simulink model "sim_explicit_IC_nonlinear"  (R2020b)
settings: Solver=VariableStepAuto  StartTime=0.0  StopTime=tsim  RelTol=1e-3
values from neighbouring files (symbols this model uses):
  g = 9.81    [init_sim.m]
  m = 0.03    [init_sim.m]
  Ts = 1e-2    (= 0.01)    [init_sim.m]
  u_max = [f_max; tau_max]    [init_sim.m]
  u_min = [f_min; tau_min]    [init_sim.m]
  x0 = zeros(6,1)    [get_sim_data.m]    (also in get_sim_data_mpc_phi.m; get_sim_data_mpc_y.m; get_sim_data_mpc_z.m; init_sim.m = 0.9*[InvSet_y.V(i,1)'; InvSet_z.V(j,1)'; InvSet_phi.V(k,1)';)
  x_max = [y_max;z_max;angle_max;vy_max;vz_max;arate_max]    [init_sim.m]
  x_min = [y_min;z_min;angle_min;vy_min;vz_min;arate_min]    [init_sim.m]
undefined symbols (not defined in the file or in its folder): pid_att, quad_ic_y, quad_ic_z, uavPlanarNonlin
libraries: pid_lib x1
settings Model: SimulationMode=accelerator  Creator=zboucek  LastModifiedBy=zboucek
settings DataIOCC: ReturnWorkspaceOutputs=off
settings DebuggingCC: ArithmeticOperatorsInVariantConditions=warning
settings SFSimCC: SimUseLocalCustomCode=off  CustomCodeUndefinedFunction=UseInterfaceOnly
settings RTWCC: RTWUseLocalCustomCode=off

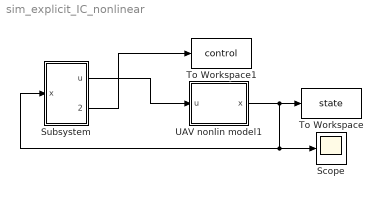
== system sim_explicit_IC_nonlinear ==
  Scope : Scope
  Subsystem : Subsystem
  To Workspace : ToWorkspace  VariableName=state  SaveFormat=Structure With Time  SampleTime=Ts
  To Workspace1 : ToWorkspace  VariableName=control  SaveFormat=Structure With Time  SampleTime=Ts
  UAV nonlin model1 : Subsystem
  wires:
  UAV nonlin model1/1(x) -> Scope/1, Subsystem/1(x), To Workspace/1
  Subsystem/1(u) -> UAV nonlin model1/1(u)
  Subsystem/2(u_ctrl) -> To Workspace1/1

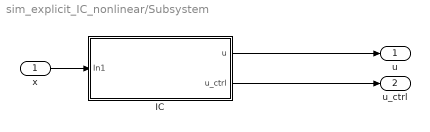
== system sim_explicit_IC_nonlinear/Subsystem ==
  x : Inport
  IC : Subsystem
  u : Outport  VectorParamsAs1DForOutWhenUnconnected=off
  u_ctrl : Outport  Port=2  VectorParamsAs1DForOutWhenUnconnected=off
  wires:
  x/1 -> IC/1(In1)
  IC/1(u) -> u/1
  IC/2(u_ctrl) -> u_ctrl/1

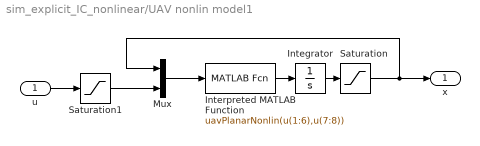
== system sim_explicit_IC_nonlinear/UAV nonlin model1 ==
  u : Inport
  Integrator : Integrator  InitialCondition=x0
  Interpreted MATLAB Function : MATLABFcn  MATLABFcn=uavPlanarNonlin(u(1:6),u(7:8))  OutputDimensions=6
  Mux : Mux  Inputs=2
  Saturation : Saturate  UpperLimit=x_max  LowerLimit=x_min
  Saturation1 : Saturate  UpperLimit=u_max  LowerLimit=u_min
  x : Outport  VectorParamsAs1DForOutWhenUnconnected=off
  wires:
  Mux/1 -> Interpreted MATLAB Function/1
  Interpreted MATLAB Function/1 -> Integrator/1
  u/1 -> Saturation1/1
  Integrator/1 -> Saturation/1
  Saturation/1 -> Mux/1, x/1
  Saturation1/1 -> Mux/2

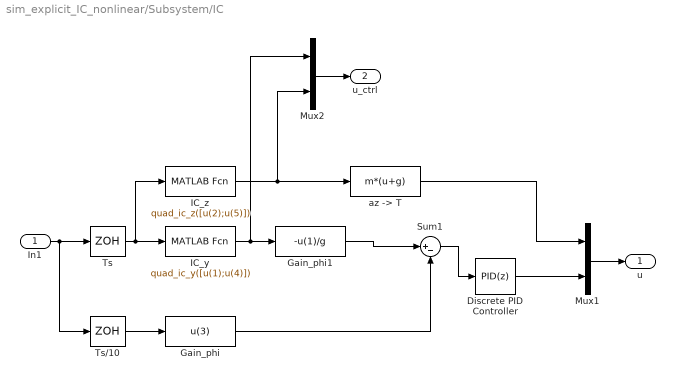
== system sim_explicit_IC_nonlinear/Subsystem/IC ==
  In1 : Inport
  Discrete PID Controller : pid_lib/PID Controller  Controller=PID  Form=Parallel  TimeDomain=Discrete-time  UseExternalTs=off  SampleTime=Ts/10  IntegratorMethod=Forward Euler  FilterMethod=Forward Euler  ControllerParametersSource=internal  P=pid_att.Kp  I=pid_att.Ki  D=pid_att.Kd  UseFilter=on  N=100  TunerSelectOption=Transfer Function Based (PID Tuner App)  InitialConditionSource=internal  InitialConditionForIntegrator=0  InitialConditionForFilter=0  DifferentiatorICPrevScaledInput=0  ExternalReset=none  TrackingMode=off  Kt=1  LimitOutput=off  SatLimitsSource=internal  UpperSaturationLimit=inf  LowerSaturationLimit=-inf  LinearizeAsGain=off  AntiWindupMode=none  Kb=1  POutMin=[]  POutMax=[]  IOutMin=[]  IOutMax=[]  DOutMin=[]  DOutMax=[]  NOutMin=[]  NOutMax=[]  SumOutMin=[]  SumOutMax=[]  SaturationOutMin=[]  SaturationOutMax=[]  PParamMin=[]  PParamMax=[]  IParamMin=[]  IParamMax=[]  DParamMin=[]  DParamMax=[]  NParamMin=[]  NParamMax=[]  KbParamMin=[]  KbParamMax=[]  KtParamMin=[]  KtParamMax=[]  KbOutMin=[]  KbOutMax=[]  KtOutMin=[]  KtOutMax=[]  IntegratorOutMin=[]  IntegratorOutMax=[]  FilterOutMin=[]  FilterOutMax=[]  SumI1OutMin=[]  SumI1OutMax=[]  SumI2OutMin=[]  SumI2OutMax=[]  SumI3OutMin=[]  SumI3OutMax=[]  SumI4OutMin=[]  SumI4OutMax=[]  SumDOutMin=[]  SumDOutMax=[]  DifferentiatorOutMin=[]  DifferentiatorOutMax=[]  FilterDiffOutCoefMin=[]  FilterDiffOutCoefMax=[]  ReciprocalOutMin=[]  ReciprocalOutMax=[]  SumDenOutMin=[]  SumDenOutMax=[]  SumNumOutMin=[]  SumNumOutMax=[]  DivideOutMin=[]  DivideOutMax=[]  UdiffTsProdOutMin=[]  UdiffTsProdOutMax=[]  NTsProdOutMin=[]  NTsProdOutMax=[]  UintegralTsProdOutMin=[]  UintegralTsProdOutMax=[]  UngainTsProdOutMin=[]  UngainTsProdOutMax=[]  IntegratorContinuousStateAttributes=''  IntegratorStateMustResolveToSignalObject=off  IntegratorRTWStateStorageClass=Auto  FilterContinuousStateAttributes=''  FilterStateMustResolveToSignalObject=off  FilterRTWStateStorageClass=Auto  ParallelPVariant=InternalParameters  IdealPVariant=Disabled  IVariant=InternalParameters  DVariant=InternalParameters  IntegratorVariant=Discrete  SatVariant=Disabled  AWVariant=Passthrough  PCopyVariant=Disabled  TRVariant=Disabled  FdbkBlocksVariant=Forward  IdealPFdbkVariant=Disabled  SatFdbkVariant=Disabled  DerivativeFilterVariant=ForwardEulerFilter  NVariant=InternalParameters  NCopyVariant=Disabled  FilterICVariant=InternalICsFilter  IntegratorICVariant=InternalICs  ExternalResetVariant=Disabled  TRSumVariant=Passthrough  SumFdbkVariant=Disabled  SumVariant=Sum_PID  TsampFilterVariant=InternalTs  TsampNgainVariant=Passthrough  TsampIntegralVariant=Passthrough  ExternalSaturationOutDataTypeStr=Inherit: Same as second input
  Gain_phi : MATLABFcn  MATLABFcn=u(3)
  Gain_phi1 : MATLABFcn  MATLABFcn=-u(1)/g
  IC_y : MATLABFcn  MATLABFcn=quad_ic_y([u(1);u(4)])
  IC_z : MATLABFcn  MATLABFcn=quad_ic_z([u(2);u(5)])
  Mux1 : Mux  Inputs=2
  Mux2 : Mux  Inputs=2
  Sum1 : Sum  Inputs=|+-
  Ts : ZeroOrderHold  SampleTime=Ts
  Ts/10 : ZeroOrderHold  SampleTime=Ts*0.1
  "az -> T" : MATLABFcn  MATLABFcn=m*(u+g)
  u : Outport  VectorParamsAs1DForOutWhenUnconnected=off
  u_ctrl : Outport  Port=2  VectorParamsAs1DForOutWhenUnconnected=off
  wires:
  In1/1 -> Ts/10/1, Ts/1
  Ts/1 -> IC_z/1, IC_y/1
  Ts/10/1 -> Gain_phi/1
  Discrete PID Controller/1 -> Mux1/2
  IC_z/1 -> Mux2/2, "az -> T"/1
  Mux1/1 -> u/1
  IC_y/1 -> Mux2/1, Gain_phi1/1
  Sum1/1 -> Discrete PID Controller/1
  Gain_phi/1 -> Sum1/2
  Gain_phi1/1 -> Sum1/1
  "az -> T"/1 -> Mux1/1
  Mux2/1 -> u_ctrl/1
